simulink model "Model_2Systems_Manipulators"  (R2018b)
settings: Solver=ode23tb  StartTime=0.0  StopTime=10  RelTol=1e-3
values from neighbouring files (symbols this model uses):
  KL = [H_L1*TL(1:2,1:2) -H_L1 ; TL(3:4,1:2)+TL(3:4,3:4)*H_L1*TL(1:2,1:2) -TL(3:4,3:4)*H_L1]    [LaplaceScattering.m]    (also in SetScatteringGain.m)
  KR = [H_R1*TR(1:2,1:2) -H_R1 ; TR(3:4,1:2)+TR(3:4,3:4)*H_R1*TR(1:2,1:2) -TR(3:4,3:4)*H_R1]    [LaplaceScattering.m]    (also in SetScatteringGain.m)
  Kv = 0*eye(2)    [Parameters.m]
  p01 = zeros(SInfo1.n, 1)    [Parameters.m]
  p02 = zeros(SInfo2.n, 1)    [Parameters.m]
  q01 = [-pi;0.2;0.4]    [Parameters.m]
  q02 = [0.5; 1.5; pi/2+pi/4]    [Parameters.m]
  T12 = T    (= 0.1)    [Parameters.m]
  T21 = T*5    (= 0.5)    [Parameters.m]
  Vr0 = 0    [Parameters.m]
undefined symbols (not defined in the file or in its folder): Simulation
settings Model: Creator=oscar  LastModifiedBy=oscar
settings SolverCC: ZeroCrossAlgorithm=Adaptive
settings DataIOCC: OutputOption=SpecifiedOutputTimes  OutputTimes=t_out
settings SFSimCC: SimUseLocalCustomCode=off
settings RTWCC: RTWUseLocalCustomCode=off

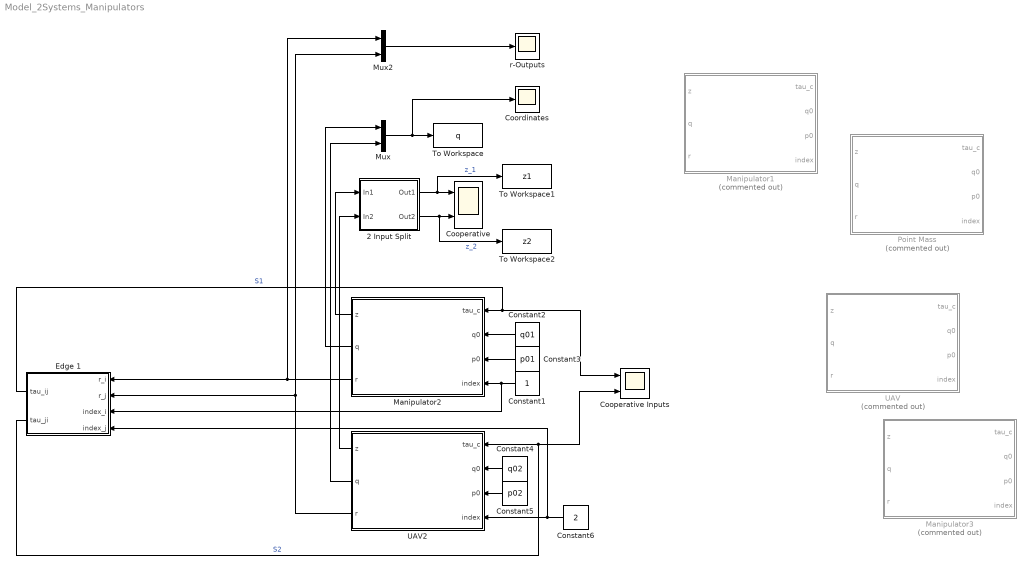
== system Model_2Systems_Manipulators ==
  2 Input Split : Subsystem
  Constant1 : Constant
  Constant2 : Constant  Value=q01
  Constant3 : Constant  Value=p01
  Constant4 : Constant  Value=q02
  Constant5 : Constant  Value=p02
  Constant6 : Constant  Value=2
  Cooperative : Scope  NumInputPorts=2
  Cooperative Inputs : Scope  NumInputPorts=2
  Coordinates : Scope
  Edge 1 : Subsystem
  Manipulator1 : Subsystem  Commented=on
  Manipulator2 : Subsystem
  Manipulator3 : Subsystem  Commented=on
  Mux : Mux  Inputs=2
  Mux2 : Mux  Inputs=2
  Point Mass : Subsystem  Commented=on
  To Workspace : ToWorkspace  VariableName=q  SaveFormat=Timeseries  SampleTime=-1
  To Workspace1 : ToWorkspace  VariableName=z1  SaveFormat=Timeseries  SampleTime=-1
  To Workspace2 : ToWorkspace  VariableName=z2  SaveFormat=Timeseries  SampleTime=-1
  UAV : Subsystem  Commented=on
  UAV2 : Subsystem
  r-Outputs : Scope
  wires:
  Mux/1 -> Coordinates/1, To Workspace/1
  Manipulator2/2(q) -> Mux/1
  UAV2/2(q) -> Mux/2
  Constant2/1 -> Manipulator2/2(q0)
  Constant3/1 -> Manipulator2/3(p0)
  Constant4/1 -> UAV2/2(q0)
  Constant5/1 -> UAV2/3(p0)
  Edge 1/1(tau_ij) -> Cooperative Inputs/1, Manipulator2/1(tau_c)  "S1"
  Edge 1/2(tau_ji) -> UAV2/1(tau_c), Cooperative Inputs/2  "S2"
  UAV2/3(r) -> Edge 1/2(r_j), Mux2/2
  Constant1/1 -> Manipulator2/4(index), Edge 1/3(index_i)
  Constant6/1 -> UAV2/4(index), Edge 1/4(index_j)
  Manipulator2/3(r) -> Edge 1/1(r_i), Mux2/1
  Mux2/1 -> r-Outputs/1
  Manipulator2/1(z) -> 2 Input Split/1(In1)
  UAV2/1(z) -> 2 Input Split/2(In2)
  2 Input Split/1(Out1) -> To Workspace1/1, Cooperative/1  "z_1"
  2 Input Split/2(Out2) -> To Workspace2/1, Cooperative/2  "z_2"

== system Model_2Systems_Manipulators/2 Input Split ==
  In1 : Inport
  In2 : Inport  Port=2
  Demux : Demux  Outputs=2
  Demux1 : Demux  Outputs=2
  Mux1 : Mux  Inputs=2
  Mux3 : Mux  Inputs=2
  Out1 : Outport
  Out2 : Outport  Port=2
  wires:
  Demux/1 -> Mux1/1
  Mux1/1 -> Out1/1
  In1/1 -> Demux/1
  Demux1/2 -> Mux3/2
  Mux3/1 -> Out2/1
  Demux1/1 -> Mux1/2
  Demux/2 -> Mux3/1
  In2/1 -> Demux1/1

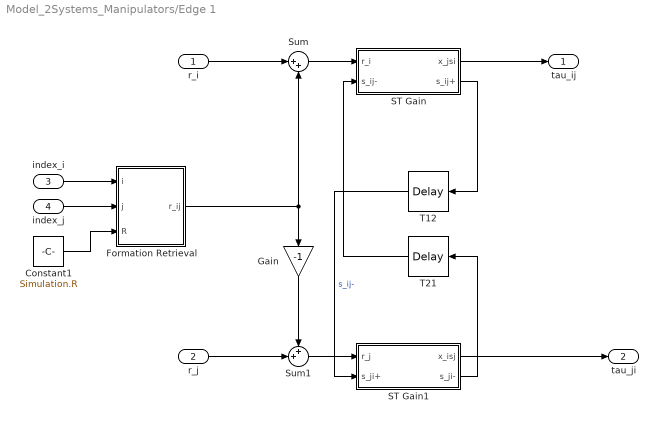
== system Model_2Systems_Manipulators/Edge 1 ==
  r_i : Inport
  r_j : Inport  Port=2
  index_i : Inport  Port=3
  index_j : Inport  Port=4
  Constant1 : Constant  Value=Simulation.R
  Formation Retrieval : MATLAB Function  TreatAsAtomicUnit=on
  Gain : Gain  Gain=-1
  ST Gain : Subsystem
  ST Gain1 : Subsystem
  Sum : Sum  Inputs=|++
  Sum1 : Sum  Inputs=++|
  T12 : TransportDelay  DelayTime=T12
  T21 : TransportDelay  DelayTime=T21
  tau_ij : Outport
  tau_ji : Outport  Port=2
  wires:
  r_i/1 -> Sum/1
  r_j/1 -> Sum1/2
  ST Gain/2(s_ij+) -> T12/1
  T21/1 -> ST Gain/2(s_ij-)
  T12/1 -> ST Gain1/2(s_ji+)  "s_ij-"
  ST Gain1/2(s_ji-) -> T21/1
  ST Gain/1(x_jsi) -> tau_ij/1
  ST Gain1/1(x_isj) -> tau_ji/1
  Sum/1 -> ST Gain/1(r_i)
  Sum1/1 -> ST Gain1/1(r_j)
  index_i/1 -> Formation Retrieval/1(i)
  index_j/1 -> Formation Retrieval/2(j)
  Formation Retrieval/1(r_ij) -> Gain/1, Sum/2
  Gain/1 -> Sum1/1
  Constant1/1 -> Formation Retrieval/3(R)

== system Model_2Systems_Manipulators/Manipulator1 ==
  tau_c : Inport
  q0 : Inport  Port=2
  p0 : Inport  Port=3
  index : Inport  Port=4
  Hamiltonian Plant : Subsystem
  Input Compensation : Scope  NumInputPorts=2
  Levenberg Compensation : MATLAB Function  Commented=on  TreatAsAtomicUnit=on
  Local Input : Scope
  MATLAB Function1 : MATLAB Function  TreatAsAtomicUnit=on
  Passivating Feedback : Scope
  Sum : Sum  Inputs=|++
  z : Outport
  q : Outport  Port=2
  r : Outport  Port=3
  wires:
  MATLAB Function1/1(tau) -> Hamiltonian Plant/3(tau_l), Local Input/1
  Hamiltonian Plant/4(p) -> MATLAB Function1/1(p)
  Hamiltonian Plant/3(q) -> q/1, MATLAB Function1/2(q)
  Hamiltonian Plant/5(z) -> z/1
  Hamiltonian Plant/2(r) -> r/1
  q0/1 -> Hamiltonian Plant/4(q0)
  p0/1 -> Hamiltonian Plant/5(p0)
  MATLAB Function1/2(tau_fb) -> Sum/2, Passivating Feedback/1
  index/1 -> Hamiltonian Plant/6(index), MATLAB Function1/3(index)
  Sum/1 -> Hamiltonian Plant/2(tau_c_hat), Input Compensation/2, Input Compensation/1  "tau_k"
  tau_c/1 -> Sum/1, Hamiltonian Plant/7(tau_c)  "tau_c_hat"

== system Model_2Systems_Manipulators/Manipulator2 ==
  tau_c : Inport
  q0 : Inport  Port=2
  p0 : Inport  Port=3
  index : Inport  Port=4
  Hamiltonian Plant : Subsystem
  Levenberg Compensation : MATLAB Function  Commented=on  TreatAsAtomicUnit=on
  Local Input : Scope
  MATLAB Function1 : MATLAB Function  TreatAsAtomicUnit=on
  Passivating Feedback : Scope
  Sum : Sum  Inputs=|++
  System Input : Scope
  z : Outport
  q : Outport  Port=2
  r : Outport  Port=3
  wires:
  MATLAB Function1/1(tau) -> Hamiltonian Plant/2(tau_l), Local Input/1
  Hamiltonian Plant/3(p) -> MATLAB Function1/1(p)
  Hamiltonian Plant/2(q) -> MATLAB Function1/2(q), q/1
  Hamiltonian Plant/4(z) -> z/1
  Hamiltonian Plant/1(r) -> r/1
  q0/1 -> Hamiltonian Plant/3(q0)
  p0/1 -> Hamiltonian Plant/4(p0)
  MATLAB Function1/2(tau_fb) -> Sum/2, Passivating Feedback/1
  index/1 -> Hamiltonian Plant/5(index), MATLAB Function1/3(index)
  Sum/1 -> Hamiltonian Plant/1(tau_c_hat), System Input/1  "tau_k"
  tau_c/1 -> Sum/1, Hamiltonian Plant/6(tau_c)  "tau_c_hat"

== system Model_2Systems_Manipulators/Manipulator3 ==
  note: z_dot Loop
  tau_c : Inport
  q0 : Inport  Port=2
  p0 : Inport  Port=3
  index : Inport  Port=4
  Gain : Gain  Gain=-Kv  Multiplication=Matrix(K*u)
  Hamiltonian Plant : Subsystem
  Input Compensation : Scope  NumInputPorts=2
  Levenberg Compensation : MATLAB Function  TreatAsAtomicUnit=on
  Local Input : Scope
  MATLAB Function1 : MATLAB Function  TreatAsAtomicUnit=on
  Passivating Feedback : Scope
  Sum : Sum  Inputs=|++
  z : Outport
  q : Outport  Port=2
  r : Outport  Port=3
  wires:
  MATLAB Function1/1(tau) -> Hamiltonian Plant/3(tau_l), Local Input/1
  Hamiltonian Plant/4(p) -> MATLAB Function1/1(p)
  Hamiltonian Plant/3(q) -> Levenberg Compensation/1(q), q/1, MATLAB Function1/2(q)
  Hamiltonian Plant/5(z) -> z/1
  Hamiltonian Plant/2(r) -> r/1
  q0/1 -> Hamiltonian Plant/4(q0)
  p0/1 -> Hamiltonian Plant/5(p0)
  MATLAB Function1/2(tau_fb) -> Sum/2, Passivating Feedback/1
  index/1 -> Levenberg Compensation/3(index), Hamiltonian Plant/6(index), MATLAB Function1/3(index)
  Hamiltonian Plant/1(z_dot) -> Gain/1
  Sum/1 -> Levenberg Compensation/2(tau_k), Input Compensation/1  "tau_k"
  tau_c/1 -> Sum/1, Hamiltonian Plant/7(tau_c)  "tau_c_hat"
  Levenberg Compensation/1(tau_c) -> Input Compensation/2, Hamiltonian Plant/2(tau_c_hat)  "tau_c_hat"

== system Model_2Systems_Manipulators/Point Mass ==
  tau_c : Inport
  q0 : Inport  Port=2
  p0 : Inport  Port=3
  index : Inport  Port=4
  Hamiltonian Plant : Subsystem
  MATLAB Function1 : MATLAB Function  TreatAsAtomicUnit=on
  Scope : Scope
  Sum : Sum  Inputs=|++
  z : Outport
  q : Outport  Port=2
  r : Outport  Port=3
  wires:
  MATLAB Function1/1(tau) -> Hamiltonian Plant/2(tau_l)
  tau_c/1 -> Sum/1
  Hamiltonian Plant/3(p) -> MATLAB Function1/1(p)
  Hamiltonian Plant/2(q) -> MATLAB Function1/2(q), q/1
  Hamiltonian Plant/4(z) -> z/1
  Hamiltonian Plant/1(r) -> r/1
  q0/1 -> Hamiltonian Plant/3(q0)
  p0/1 -> Hamiltonian Plant/4(p0)
  MATLAB Function1/2(tau_fb) -> Scope/1, Sum/2
  Sum/1 -> Hamiltonian Plant/1(tau_c)
  index/1 -> Hamiltonian Plant/5(index), MATLAB Function1/3(index)

== system Model_2Systems_Manipulators/UAV ==
  tau_c : Inport
  q0 : Inport  Port=2
  p0 : Inport  Port=3
  index : Inport  Port=4
  Gain : Gain  Gain=Kv  Multiplication=Matrix(K*u)
  Hamiltonian Plant : Subsystem
  MATLAB Function1 : MATLAB Function  TreatAsAtomicUnit=on
  Scope : Scope
  Scope1 : Scope
  Sum : Sum  Inputs=|++
  Sum1 : Sum  Inputs=-+|
  z : Outport
  q : Outport  Port=2
  r : Outport  Port=3
  wires:
  MATLAB Function1/1(tau) -> Scope1/1, Hamiltonian Plant/2(tau_l)
  tau_c/1 -> Sum/1
  Hamiltonian Plant/3(p) -> MATLAB Function1/1(p)
  Hamiltonian Plant/2(q) -> MATLAB Function1/2(q), q/1
  Hamiltonian Plant/4(z) -> z/1
  Hamiltonian Plant/1(r) -> r/1
  q0/1 -> Hamiltonian Plant/3(q0)
  p0/1 -> Hamiltonian Plant/4(p0)
  MATLAB Function1/2(tau_fb) -> Scope/1, Sum/2
  Sum/1 -> Sum1/2
  index/1 -> Hamiltonian Plant/5(index), MATLAB Function1/3(index)
  Hamiltonian Plant/5(y) -> Gain/1
  Sum1/1 -> Hamiltonian Plant/1(tau_c)
  Gain/1 -> Sum1/1

== system Model_2Systems_Manipulators/UAV2 ==
  tau_c : Inport
  q0 : Inport  Port=2
  p0 : Inport  Port=3
  index : Inport  Port=4
  Hamiltonian Plant : Subsystem
  Levenberg Compensation : MATLAB Function  Commented=on  TreatAsAtomicUnit=on
  Local Input : Scope
  MATLAB Function : MATLAB Function  TreatAsAtomicUnit=on
  MATLAB Function1 : MATLAB Function  Commented=on  TreatAsAtomicUnit=on
  Passivating Feedback : Scope
  Sum : Sum  Inputs=|++
  System Input : Scope
  z : Outport
  q : Outport  Port=2
  r : Outport  Port=3
  wires:
  ? -> Hamiltonian Plant/2(tau_l), Local Input/1
  Hamiltonian Plant/3(p) -> ?
  Hamiltonian Plant/2(q) -> q/1
  Hamiltonian Plant/4(z) -> z/1
  Hamiltonian Plant/1(r) -> r/1
  q0/1 -> Hamiltonian Plant/3(q0)
  p0/1 -> Hamiltonian Plant/4(p0)
  ? -> Sum/2, Passivating Feedback/1
  index/1 -> Hamiltonian Plant/5(index)
  Sum/1 -> Hamiltonian Plant/1(tau_c_hat), System Input/1  "tau_c_hat"
  tau_c/1 -> Sum/1, Hamiltonian Plant/6(tau_c)

== system Model_2Systems_Manipulators/Edge 1/ST Gain ==
  r_i : Inport
  s_ij- : Inport  Port=2
  Demux : Demux  Outputs=2
  Gain : Gain  Gain=KL  Multiplication=Matrix(K*u)
  Mux : Mux  Inputs=2
  x_jsi : Outport
  s_ij+ : Outport  Port=2
  wires:
  s_ij-/1 -> Mux/1
  r_i/1 -> Mux/2
  Mux/1 -> Gain/1
  Gain/1 -> Demux/1
  Demux/1 -> x_jsi/1
  Demux/2 -> s_ij+/1

== system Model_2Systems_Manipulators/Edge 1/ST Gain1 ==
  r_j : Inport
  s_ji+ : Inport  Port=2
  Demux : Demux  Outputs=2
  Gain : Gain  Gain=KR  Multiplication=Matrix(K*u)
  Mux : Mux  Inputs=2
  x_isj : Outport
  s_ji- : Outport  Port=2
  wires:
  s_ji+/1 -> Mux/1
  r_j/1 -> Mux/2
  Mux/1 -> Gain/1
  Gain/1 -> Demux/1
  Demux/1 -> x_isj/1
  Demux/2 -> s_ji-/1

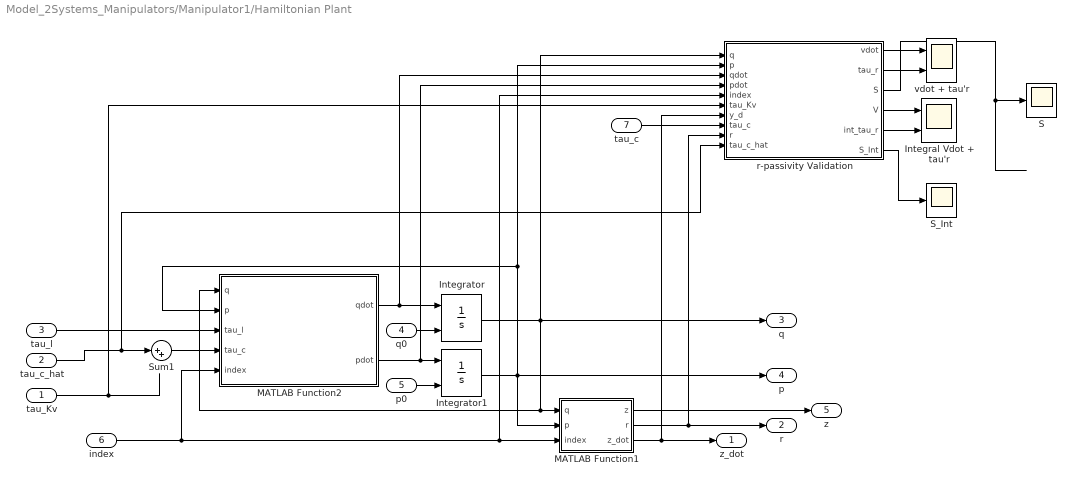
== system Model_2Systems_Manipulators/Manipulator1/Hamiltonian Plant ==
  tau_Kv : Inport
  tau_c_hat : Inport  Port=2
  tau_l : Inport  Port=3
  q0 : Inport  Port=4
  p0 : Inport  Port=5
  index : Inport  Port=6
  tau_c : Inport  Port=7
  Integral Vdot + tau'r : Scope  NumInputPorts=2
  Integrator : Integrator  InitialConditionSource=external  InitialCondition=q01
  Integrator1 : Integrator  InitialConditionSource=external  InitialCondition=p02
  MATLAB Function1 : MATLAB Function  TreatAsAtomicUnit=on
  MATLAB Function2 : MATLAB Function  TreatAsAtomicUnit=on
  S : Scope
  S_Int : Scope
  Sum1 : Sum  Inputs=|++
  r-passivity Validation : Subsystem
  vdot + tau'r : Scope  NumInputPorts=2
  z_dot : Outport
  r : Outport  Port=2
  q : Outport  Port=3
  p : Outport  Port=4
  z : Outport  Port=5
  wires:
  tau_l/1 -> MATLAB Function2/3(tau_l)
  MATLAB Function2/2(pdot) -> r-passivity Validation/4(pdot), Integrator1/1
  Integrator1/1 -> r-passivity Validation/2(p), MATLAB Function2/2(p), p/1, MATLAB Function1/2(p)
  Integrator/1 -> r-passivity Validation/1(q), q/1, MATLAB Function2/1(q), MATLAB Function1/1(q)
  MATLAB Function2/1(qdot) -> r-passivity Validation/3(qdot), Integrator/1
  p0/1 -> Integrator1/2
  tau_c_hat/1 -> r-passivity Validation/10(tau_c_hat), Sum1/1
  q0/1 -> Integrator/2
  MATLAB Function1/1(z) -> z/1
  MATLAB Function1/2(r) -> r-passivity Validation/9(r), r/1
  index/1 -> r-passivity Validation/5(index), MATLAB Function1/3(index), MATLAB Function2/5(index)
  MATLAB Function1/3(z_dot) -> r-passivity Validation/7(y_d), z_dot/1
  r-passivity Validation/1(vdot) -> vdot + tau'r/1
  r-passivity Validation/2(tau_r) -> vdot + tau'r/2
  r-passivity Validation/5(int_tau_r) -> Integral Vdot + tau'r/2
  r-passivity Validation/4(V) -> Integral Vdot + tau'r/1
  r-passivity Validation/3(S) -> S/1
  tau_c/1 -> r-passivity Validation/8(tau_c)
  tau_Kv/1 -> r-passivity Validation/6(tau_Kv)
  Sum1/1 -> MATLAB Function2/4(tau_c)
  r-passivity Validation/6(S_Int) -> S_Int/1

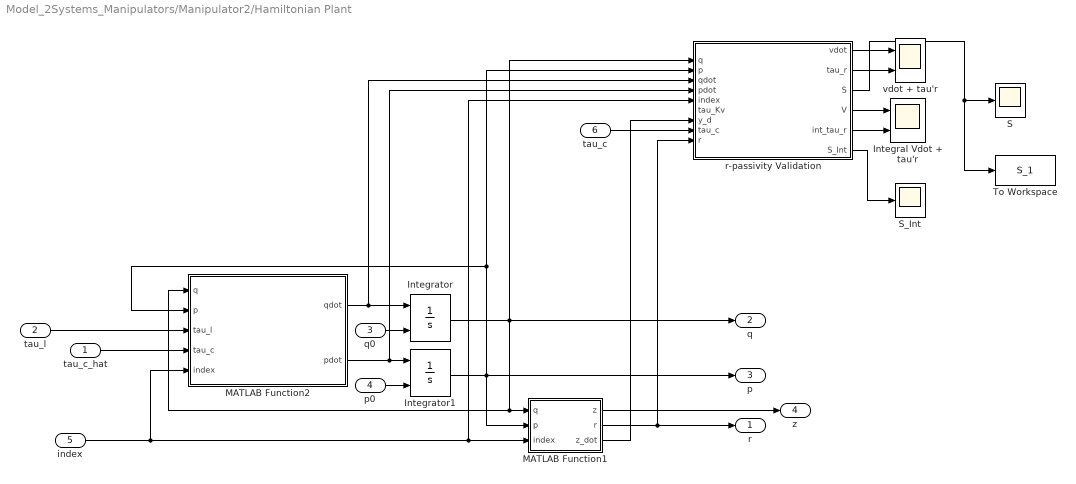
== system Model_2Systems_Manipulators/Manipulator2/Hamiltonian Plant ==
  tau_c_hat : Inport
  tau_l : Inport  Port=2
  q0 : Inport  Port=3
  p0 : Inport  Port=4
  index : Inport  Port=5
  tau_c : Inport  Port=6
  Integral Vdot + tau'r : Scope  NumInputPorts=2
  Integrator : Integrator  InitialConditionSource=external  InitialCondition=q01
  Integrator1 : Integrator  InitialConditionSource=external  InitialCondition=p02
  MATLAB Function1 : MATLAB Function  TreatAsAtomicUnit=on
  MATLAB Function2 : MATLAB Function  TreatAsAtomicUnit=on
  S : Scope
  S_Int : Scope
  To Workspace : ToWorkspace  VariableName=S_1  SaveFormat=Timeseries  SampleTime=-1
  r-passivity Validation : Subsystem
  vdot + tau'r : Scope  NumInputPorts=2
  r : Outport
  q : Outport  Port=2
  p : Outport  Port=3
  z : Outport  Port=4
  wires:
  tau_l/1 -> MATLAB Function2/3(tau_l)
  MATLAB Function2/2(pdot) -> r-passivity Validation/4(pdot), Integrator1/1
  Integrator1/1 -> r-passivity Validation/2(p), MATLAB Function2/2(p), p/1, MATLAB Function1/2(p)
  Integrator/1 -> r-passivity Validation/1(q), q/1, MATLAB Function2/1(q), MATLAB Function1/1(q)
  MATLAB Function2/1(qdot) -> r-passivity Validation/3(qdot), Integrator/1
  p0/1 -> Integrator1/2
  q0/1 -> Integrator/2
  MATLAB Function1/1(z) -> z/1
  MATLAB Function1/2(r) -> r-passivity Validation/9(r), r/1
  index/1 -> r-passivity Validation/5(index), MATLAB Function1/3(index), MATLAB Function2/5(index)
  MATLAB Function1/3(z_dot) -> r-passivity Validation/7(y_d)
  r-passivity Validation/1(vdot) -> vdot + tau'r/1
  r-passivity Validation/2(tau_r) -> vdot + tau'r/2
  r-passivity Validation/5(int_tau_r) -> Integral Vdot + tau'r/2
  r-passivity Validation/4(V) -> Integral Vdot + tau'r/1
  r-passivity Validation/3(S) -> To Workspace/1, S/1
  tau_c/1 -> r-passivity Validation/8(tau_c)
  tau_c_hat/1 -> MATLAB Function2/4(tau_c)
  r-passivity Validation/6(S_Int) -> S_Int/1

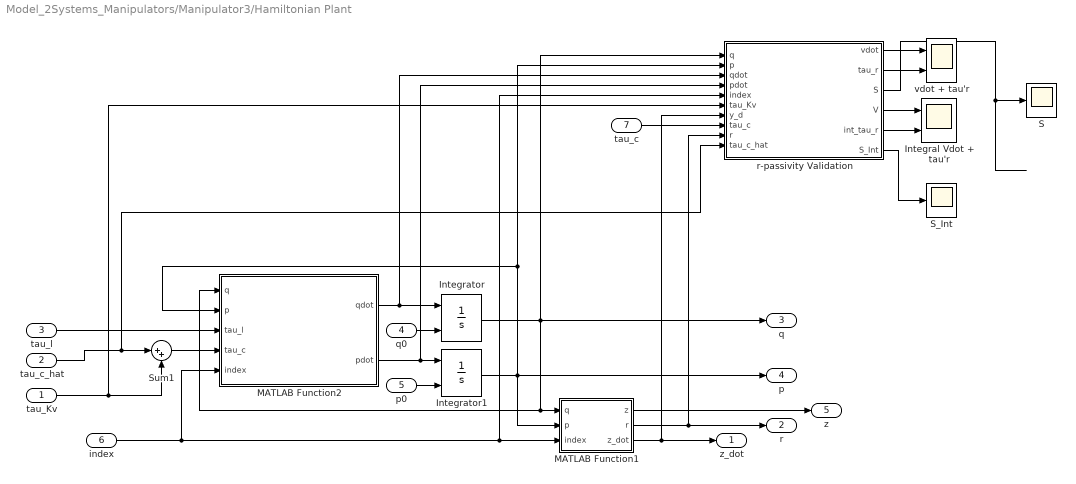
== system Model_2Systems_Manipulators/Manipulator3/Hamiltonian Plant ==
  tau_Kv : Inport
  tau_c_hat : Inport  Port=2
  tau_l : Inport  Port=3
  q0 : Inport  Port=4
  p0 : Inport  Port=5
  index : Inport  Port=6
  tau_c : Inport  Port=7
  Integral Vdot + tau'r : Scope  NumInputPorts=2
  Integrator : Integrator  InitialConditionSource=external  InitialCondition=q01
  Integrator1 : Integrator  InitialConditionSource=external  InitialCondition=p02
  MATLAB Function1 : MATLAB Function  TreatAsAtomicUnit=on
  MATLAB Function2 : MATLAB Function  TreatAsAtomicUnit=on
  S : Scope
  S_Int : Scope
  Sum1 : Sum  Inputs=|++
  r-passivity Validation : Subsystem
  vdot + tau'r : Scope  NumInputPorts=2
  z_dot : Outport
  r : Outport  Port=2
  q : Outport  Port=3
  p : Outport  Port=4
  z : Outport  Port=5
  wires:
  tau_l/1 -> MATLAB Function2/3(tau_l)
  MATLAB Function2/2(pdot) -> r-passivity Validation/4(pdot), Integrator1/1
  Integrator1/1 -> r-passivity Validation/2(p), MATLAB Function2/2(p), p/1, MATLAB Function1/2(p)
  Integrator/1 -> r-passivity Validation/1(q), q/1, MATLAB Function2/1(q), MATLAB Function1/1(q)
  MATLAB Function2/1(qdot) -> r-passivity Validation/3(qdot), Integrator/1
  p0/1 -> Integrator1/2
  tau_c_hat/1 -> r-passivity Validation/10(tau_c_hat), Sum1/1
  q0/1 -> Integrator/2
  MATLAB Function1/1(z) -> z/1
  MATLAB Function1/2(r) -> r-passivity Validation/9(r), r/1
  index/1 -> r-passivity Validation/5(index), MATLAB Function1/3(index), MATLAB Function2/5(index)
  MATLAB Function1/3(z_dot) -> r-passivity Validation/7(y_d), z_dot/1
  r-passivity Validation/1(vdot) -> vdot + tau'r/1
  r-passivity Validation/2(tau_r) -> vdot + tau'r/2
  r-passivity Validation/5(int_tau_r) -> Integral Vdot + tau'r/2
  r-passivity Validation/4(V) -> Integral Vdot + tau'r/1
  r-passivity Validation/3(S) -> S/1
  tau_c/1 -> r-passivity Validation/8(tau_c)
  tau_Kv/1 -> Sum1/2, r-passivity Validation/6(tau_Kv)
  Sum1/1 -> MATLAB Function2/4(tau_c)
  r-passivity Validation/6(S_Int) -> S_Int/1

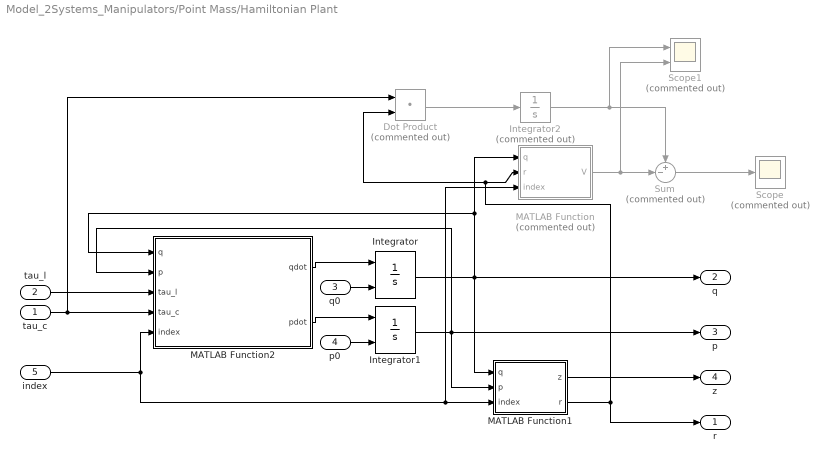
== system Model_2Systems_Manipulators/Point Mass/Hamiltonian Plant ==
  tau_c : Inport
  tau_l : Inport  Port=2
  q0 : Inport  Port=3
  p0 : Inport  Port=4
  index : Inport  Port=5
  Dot Product : DotProduct  Commented=on  InputSameDT=on  OutDataTypeStr=Inherit: Inherit via internal rule
  Integrator : Integrator  InitialConditionSource=external  InitialCondition=q01
  Integrator1 : Integrator  InitialConditionSource=external  InitialCondition=p02
  Integrator2 : Integrator  Commented=on
  MATLAB Function : MATLAB Function  Commented=on  TreatAsAtomicUnit=on
  MATLAB Function1 : MATLAB Function  TreatAsAtomicUnit=on
  MATLAB Function2 : MATLAB Function  TreatAsAtomicUnit=on
  Scope : Scope  Commented=on
  Scope1 : Scope  Commented=on  NumInputPorts=2
  Sum : Sum  Commented=on  Inputs=+-|
  r : Outport
  q : Outport  Port=2
  p : Outport  Port=3
  z : Outport  Port=4
  wires:
  tau_l/1 -> MATLAB Function2/3(tau_l)
  MATLAB Function2/2(pdot) -> Integrator1/1
  Integrator1/1 -> MATLAB Function1/2(p), MATLAB Function2/2(p), p/1
  Integrator/1 -> MATLAB Function1/1(q), MATLAB Function/1(q), MATLAB Function2/1(q), q/1
  MATLAB Function2/1(qdot) -> Integrator/1
  p0/1 -> Integrator1/2
  tau_c/1 -> MATLAB Function2/4(tau_c), Dot Product/1
  q0/1 -> Integrator/2
  MATLAB Function/1(V) -> Scope1/2, Sum/2
  Dot Product/1 -> Integrator2/1
  Sum/1 -> Scope/1
  Integrator2/1 -> Scope1/1, Sum/1
  MATLAB Function1/1(z) -> z/1
  MATLAB Function1/2(r) -> MATLAB Function/2(r), Dot Product/2, r/1
  index/1 -> MATLAB Function/3(index), MATLAB Function1/3(index), MATLAB Function2/5(index)

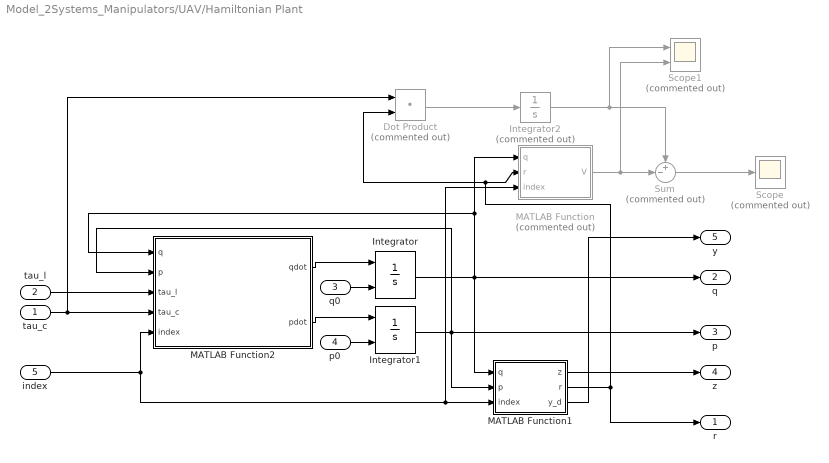
== system Model_2Systems_Manipulators/UAV/Hamiltonian Plant ==
  tau_c : Inport
  tau_l : Inport  Port=2
  q0 : Inport  Port=3
  p0 : Inport  Port=4
  index : Inport  Port=5
  Dot Product : DotProduct  Commented=on  InputSameDT=on  OutDataTypeStr=Inherit: Inherit via internal rule
  Integrator : Integrator  InitialConditionSource=external  InitialCondition=q01
  Integrator1 : Integrator  InitialConditionSource=external  InitialCondition=p02
  Integrator2 : Integrator  Commented=on
  MATLAB Function : MATLAB Function  Commented=on  TreatAsAtomicUnit=on
  MATLAB Function1 : MATLAB Function  TreatAsAtomicUnit=on
  MATLAB Function2 : MATLAB Function  TreatAsAtomicUnit=on
  Scope : Scope  Commented=on
  Scope1 : Scope  Commented=on  NumInputPorts=2
  Sum : Sum  Commented=on  Inputs=+-|
  r : Outport
  q : Outport  Port=2
  p : Outport  Port=3
  z : Outport  Port=4
  y : Outport  Port=5
  wires:
  tau_l/1 -> MATLAB Function2/3(tau_l)
  MATLAB Function2/2(pdot) -> Integrator1/1
  Integrator1/1 -> MATLAB Function1/2(p), MATLAB Function2/2(p), p/1
  Integrator/1 -> MATLAB Function1/1(q), MATLAB Function/1(q), MATLAB Function2/1(q), q/1
  MATLAB Function2/1(qdot) -> Integrator/1
  p0/1 -> Integrator1/2
  tau_c/1 -> MATLAB Function2/4(tau_c), Dot Product/1
  q0/1 -> Integrator/2
  MATLAB Function/1(V) -> Scope1/2, Sum/2
  Dot Product/1 -> Integrator2/1
  Sum/1 -> Scope/1
  Integrator2/1 -> Scope1/1, Sum/1
  MATLAB Function1/1(z) -> z/1
  MATLAB Function1/2(r) -> r/1, MATLAB Function/2(r), Dot Product/2
  index/1 -> MATLAB Function/3(index), MATLAB Function1/3(index), MATLAB Function2/5(index)
  MATLAB Function1/3(y_d) -> y/1

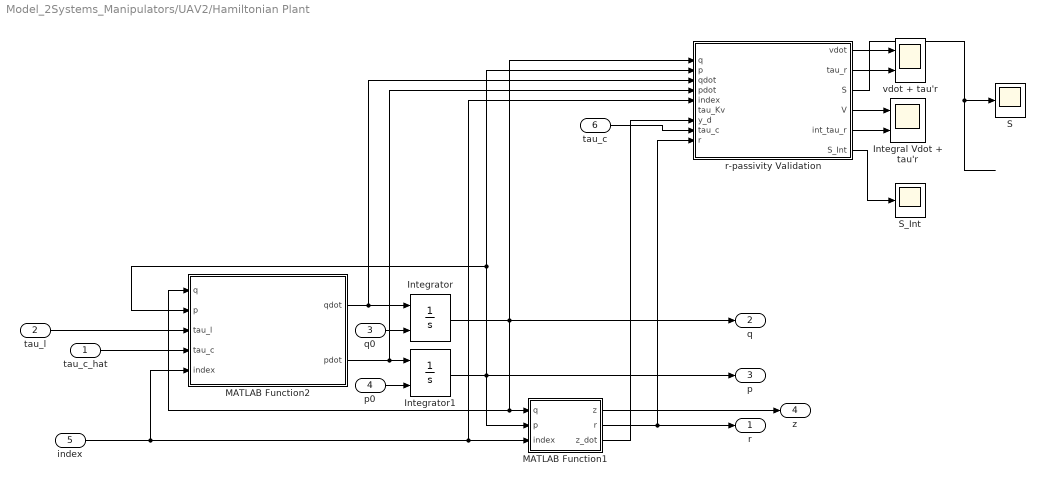
== system Model_2Systems_Manipulators/UAV2/Hamiltonian Plant ==
  tau_c_hat : Inport
  tau_l : Inport  Port=2
  q0 : Inport  Port=3
  p0 : Inport  Port=4
  index : Inport  Port=5
  tau_c : Inport  Port=6
  Integral Vdot + tau'r : Scope  NumInputPorts=2
  Integrator : Integrator  InitialConditionSource=external  InitialCondition=q01
  Integrator1 : Integrator  InitialConditionSource=external  InitialCondition=p02
  MATLAB Function1 : MATLAB Function  TreatAsAtomicUnit=on
  MATLAB Function2 : MATLAB Function  TreatAsAtomicUnit=on
  S : Scope
  S_Int : Scope
  r-passivity Validation : Subsystem
  vdot + tau'r : Scope  NumInputPorts=2
  r : Outport
  q : Outport  Port=2
  p : Outport  Port=3
  z : Outport  Port=4
  wires:
  tau_l/1 -> MATLAB Function2/3(tau_l)
  MATLAB Function2/2(pdot) -> r-passivity Validation/4(pdot), Integrator1/1
  Integrator1/1 -> r-passivity Validation/2(p), MATLAB Function2/2(p), p/1, MATLAB Function1/2(p)
  Integrator/1 -> r-passivity Validation/1(q), q/1, MATLAB Function2/1(q), MATLAB Function1/1(q)
  MATLAB Function2/1(qdot) -> r-passivity Validation/3(qdot), Integrator/1
  p0/1 -> Integrator1/2
  q0/1 -> Integrator/2
  MATLAB Function1/1(z) -> z/1
  MATLAB Function1/2(r) -> r-passivity Validation/9(r), r/1
  index/1 -> r-passivity Validation/5(index), MATLAB Function1/3(index), MATLAB Function2/5(index)
  MATLAB Function1/3(z_dot) -> r-passivity Validation/7(y_d)
  r-passivity Validation/1(vdot) -> vdot + tau'r/1
  r-passivity Validation/2(tau_r) -> vdot + tau'r/2
  r-passivity Validation/5(int_tau_r) -> Integral Vdot + tau'r/2
  r-passivity Validation/4(V) -> Integral Vdot + tau'r/1
  r-passivity Validation/3(S) -> S/1
  tau_c/1 -> r-passivity Validation/8(tau_c)
  tau_c_hat/1 -> MATLAB Function2/4(tau_c)
  r-passivity Validation/6(S_Int) -> S_Int/1

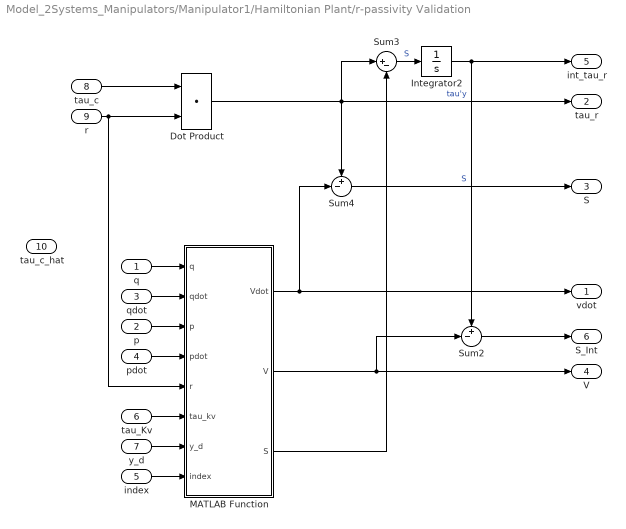
== system Model_2Systems_Manipulators/Manipulator1/Hamiltonian Plant/r-passivity Validation ==
  q : Inport
  p : Inport  Port=2
  qdot : Inport  Port=3
  pdot : Inport  Port=4
  index : Inport  Port=5
  tau_Kv : Inport  Port=6
  y_d : Inport  Port=7
  tau_c : Inport  Port=8
  r : Inport  Port=9
  tau_c_hat : Inport  Port=10
  Dot Product : DotProduct  InputSameDT=on  OutDataTypeStr=Inherit: Inherit via internal rule
  Integrator2 : Integrator
  MATLAB Function : MATLAB Function  TreatAsAtomicUnit=on
  Sum2 : Sum  Inputs=+-|
  Sum3 : Sum  Inputs=|+-
  Sum4 : Sum  Inputs=+-|
  vdot : Outport
  tau_r : Outport  Port=2
  S : Outport  Port=3
  V : Outport  Port=4
  int_tau_r : Outport  Port=5
  S_Int : Outport  Port=6
  wires:
  Sum4/1 -> S/1  "S"
  pdot/1 -> MATLAB Function/4(pdot)
  p/1 -> MATLAB Function/3(p)
  qdot/1 -> MATLAB Function/2(qdot)
  index/1 -> MATLAB Function/8(index)
  q/1 -> MATLAB Function/1(q)
  tau_Kv/1 -> MATLAB Function/6(tau_kv)
  y_d/1 -> MATLAB Function/7(y_d)
  tau_c/1 -> Dot Product/1
  r/1 -> Dot Product/2, MATLAB Function/5(r)
  Dot Product/1 -> Sum3/1, tau_r/1, Sum4/1  "tau'y"
  MATLAB Function/1(Vdot) -> Sum4/2, vdot/1
  MATLAB Function/2(V) -> Sum2/2, V/1
  Integrator2/1 -> int_tau_r/1, Sum2/1
  Sum2/1 -> S_Int/1
  MATLAB Function/3(S) -> Sum3/2
  Sum3/1 -> Integrator2/1  "S"

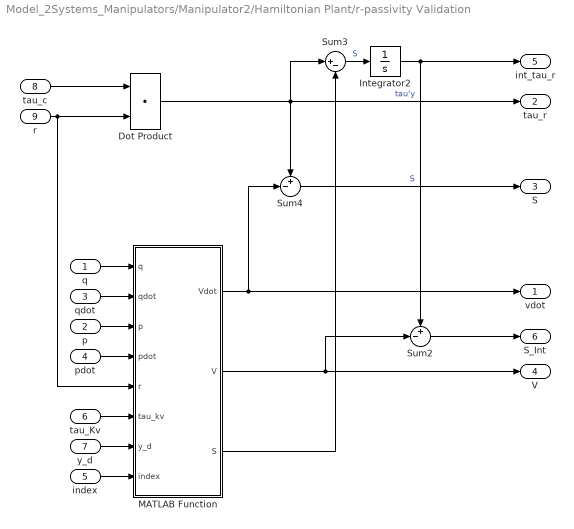
== system Model_2Systems_Manipulators/Manipulator2/Hamiltonian Plant/r-passivity Validation ==
  q : Inport
  p : Inport  Port=2
  qdot : Inport  Port=3
  pdot : Inport  Port=4
  index : Inport  Port=5
  tau_Kv : Inport  Port=6
  y_d : Inport  Port=7
  tau_c : Inport  Port=8
  r : Inport  Port=9
  Dot Product : DotProduct  InputSameDT=on  OutDataTypeStr=Inherit: Inherit via internal rule
  Integrator2 : Integrator
  MATLAB Function : MATLAB Function  TreatAsAtomicUnit=on
  Sum2 : Sum  Inputs=+-|
  Sum3 : Sum  Inputs=|+-
  Sum4 : Sum  Inputs=+-|
  vdot : Outport
  tau_r : Outport  Port=2
  S : Outport  Port=3
  V : Outport  Port=4
  int_tau_r : Outport  Port=5
  S_Int : Outport  Port=6
  wires:
  Sum4/1 -> S/1  "S"
  pdot/1 -> MATLAB Function/4(pdot)
  p/1 -> MATLAB Function/3(p)
  qdot/1 -> MATLAB Function/2(qdot)
  index/1 -> MATLAB Function/8(index)
  q/1 -> MATLAB Function/1(q)
  tau_Kv/1 -> MATLAB Function/6(tau_kv)
  y_d/1 -> MATLAB Function/7(y_d)
  tau_c/1 -> Dot Product/1
  r/1 -> Dot Product/2, MATLAB Function/5(r)
  Dot Product/1 -> Sum3/1, tau_r/1, Sum4/1  "tau'y"
  MATLAB Function/1(Vdot) -> Sum4/2, vdot/1
  MATLAB Function/2(V) -> Sum2/2, V/1
  Integrator2/1 -> int_tau_r/1, Sum2/1
  Sum2/1 -> S_Int/1
  MATLAB Function/3(S) -> Sum3/2
  Sum3/1 -> Integrator2/1  "S"

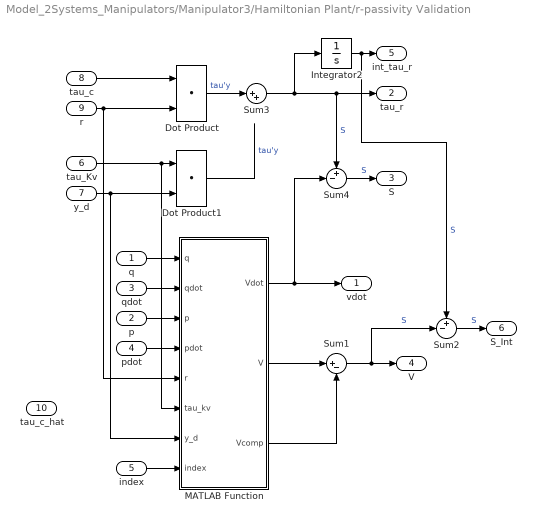
== system Model_2Systems_Manipulators/Manipulator3/Hamiltonian Plant/r-passivity Validation ==
  q : Inport
  p : Inport  Port=2
  qdot : Inport  Port=3
  pdot : Inport  Port=4
  index : Inport  Port=5
  tau_Kv : Inport  Port=6
  y_d : Inport  Port=7
  tau_c : Inport  Port=8
  r : Inport  Port=9
  tau_c_hat : Inport  Port=10
  Dot Product : DotProduct  InputSameDT=on  OutDataTypeStr=Inherit: Inherit via internal rule
  Dot Product1 : DotProduct  InputSameDT=on  OutDataTypeStr=Inherit: Inherit via internal rule
  Integrator2 : Integrator
  MATLAB Function : MATLAB Function  TreatAsAtomicUnit=on
  Sum1 : Sum  Inputs=|+-
  Sum2 : Sum  Inputs=+-|
  Sum3 : Sum  Inputs=|++
  Sum4 : Sum  Inputs=+-|
  vdot : Outport
  tau_r : Outport  Port=2
  S : Outport  Port=3
  V : Outport  Port=4
  int_tau_r : Outport  Port=5
  S_Int : Outport  Port=6
  wires:
  Sum4/1 -> S/1  "S"
  pdot/1 -> MATLAB Function/4(pdot)
  p/1 -> MATLAB Function/3(p)
  qdot/1 -> MATLAB Function/2(qdot)
  MATLAB Function/2(V) -> Sum1/1
  index/1 -> MATLAB Function/8(index)
  q/1 -> MATLAB Function/1(q)
  tau_Kv/1 -> MATLAB Function/6(tau_kv), Dot Product1/1
  y_d/1 -> Dot Product1/2, MATLAB Function/7(y_d)
  tau_c/1 -> Dot Product/1
  r/1 -> Dot Product/2, MATLAB Function/5(r)
  Dot Product/1 -> Sum3/1  "tau'y"
  Sum3/1 -> Integrator2/1, tau_r/1, Sum4/1  "S"
  Dot Product1/1 -> ?  "tau'y"
  MATLAB Function/1(Vdot) -> Sum4/2, vdot/1
  Sum1/1 -> Sum2/2, V/1  "S"
  MATLAB Function/3(Vcomp) -> Sum1/2
  Integrator2/1 -> Sum2/1, int_tau_r/1  "S"
  Sum2/1 -> S_Int/1  "S"

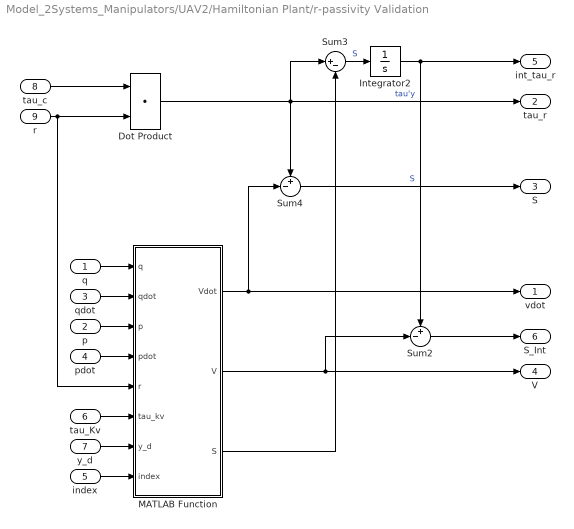
== system Model_2Systems_Manipulators/UAV2/Hamiltonian Plant/r-passivity Validation ==
  q : Inport
  p : Inport  Port=2
  qdot : Inport  Port=3
  pdot : Inport  Port=4
  index : Inport  Port=5
  tau_Kv : Inport  Port=6
  y_d : Inport  Port=7
  tau_c : Inport  Port=8
  r : Inport  Port=9
  Dot Product : DotProduct  InputSameDT=on  OutDataTypeStr=Inherit: Inherit via internal rule
  Integrator2 : Integrator
  MATLAB Function : MATLAB Function  TreatAsAtomicUnit=on
  Sum2 : Sum  Inputs=+-|
  Sum3 : Sum  Inputs=|+-
  Sum4 : Sum  Inputs=+-|
  vdot : Outport
  tau_r : Outport  Port=2
  S : Outport  Port=3
  V : Outport  Port=4
  int_tau_r : Outport  Port=5
  S_Int : Outport  Port=6
  wires:
  Sum4/1 -> S/1  "S"
  pdot/1 -> MATLAB Function/4(pdot)
  p/1 -> MATLAB Function/3(p)
  qdot/1 -> MATLAB Function/2(qdot)
  index/1 -> MATLAB Function/8(index)
  q/1 -> MATLAB Function/1(q)
  tau_Kv/1 -> MATLAB Function/6(tau_kv)
  y_d/1 -> MATLAB Function/7(y_d)
  tau_c/1 -> Dot Product/1
  r/1 -> Dot Product/2, MATLAB Function/5(r)
  Dot Product/1 -> Sum3/1, tau_r/1, Sum4/1  "tau'y"
  MATLAB Function/1(Vdot) -> Sum4/2, vdot/1
  MATLAB Function/2(V) -> Sum2/2, V/1
  Integrator2/1 -> int_tau_r/1, Sum2/1
  Sum2/1 -> S_Int/1
  MATLAB Function/3(S) -> Sum3/2
  Sum3/1 -> Integrator2/1  "S"

== matlab function Model_2Systems_Manipulators/Point Mass/Hamiltonian Plant/MATLAB Function ==
  data: q input; r input; index input; V output; Vr0 parameter
function V = fcn(q, r, index, Vr0)

%     coder.extrinsic('R_Validation');
%     V = 0;
%     [V] = R_Validation(q, r, index);
%     V = V - Vr0;
V = 0;
end

== matlab function Model_2Systems_Manipulators/Point Mass/Hamiltonian Plant/MATLAB Function1 ==
  data: q input; z output; p input; r output; index input
function [z, r] = toz(q, p, index)

    coder.extrinsic('Pointmass2D_z');
    z = zeros(2, 1);
    r = zeros(2, 1);    
    [z, r] = Pointmass2D_z(q, p, index);

== matlab function Model_2Systems_Manipulators/Manipulator2/Hamiltonian Plant/MATLAB Function1 ==
  data: q input; z output; p input; r output; index input; z_dot output
function [z, r, z_dot] = toz(q, p, index)

    coder.extrinsic('Manipulator_z');
    z = zeros(2, 1);
    r = zeros(2, 1);
    z_dot = zeros(2, 1);
    [z, r, z_dot] = Manipulator_z(q, p, index);

== matlab function Model_2Systems_Manipulators/Manipulator2/Hamiltonian Plant/MATLAB Function2 ==
  data: q input; qdot output; p input; tau_l input; pdot output; tau_c input; index input
function [qdot, pdot] = fcn(q, p, tau_l, tau_c, index)

    coder.extrinsic('Manipulator_Dynamics');
    qdot = zeros(3, 1);
    pdot = zeros(3, 1);
    [qdot, pdot] = Manipulator_Dynamics(q, p, tau_l, tau_c, index);

== matlab function Model_2Systems_Manipulators/Point Mass/Hamiltonian Plant/MATLAB Function2 ==
  data: q input; qdot output; p input; tau_l input; pdot output; tau_c input; index input
function [qdot, pdot] = fcn(q, p, tau_l, tau_c, index)

    coder.extrinsic('Pointmass2D_Dynamics');
    qdot = zeros(2, 1);
    pdot = zeros(2, 1);
    [qdot, pdot] = Pointmass2D_Dynamics(q, p, tau_l, tau_c, index);

== matlab function Model_2Systems_Manipulators/Point Mass/MATLAB Function1 ==
  data: p input; q input; tau output; tau_fb output; index input
function [tau, tau_fb] = LocalControl(p, q, index)
    

coder.extrinsic('Pointmass2D_Control');
tau = zeros(2, 1);
tau_fb = zeros(2, 1);
[tau, tau_fb] = Pointmass2D_Control(q, p, index);

== matlab function Model_2Systems_Manipulators/Manipulator1/Hamiltonian Plant/MATLAB Function1 ==
  data: q input; z output; p input; r output; index input; z_dot output
function [z, r, z_dot] = toz(q, p, index)

    coder.extrinsic('Manipulator_z');
    z = zeros(2, 1);
    r = zeros(2, 1);
    z_dot = zeros(2, 1);
    [z, r, z_dot] = Manipulator_z(q, p, index);

== matlab function Model_2Systems_Manipulators/Manipulator1/Hamiltonian Plant/MATLAB Function2 ==
  data: q input; qdot output; p input; tau_l input; pdot output; tau_c input; index input
function [qdot, pdot] = fcn(q, p, tau_l, tau_c, index)

    coder.extrinsic('Manipulator_Dynamics');
    qdot = zeros(3, 1);
    pdot = zeros(3, 1);
    [qdot, pdot] = Manipulator_Dynamics(q, p, tau_l, tau_c, index);

== matlab function Model_2Systems_Manipulators/Manipulator1/Hamiltonian Plant/r-passivity Validation/MATLAB Function ==
  data: Vdot output; q input; qdot input; p input; pdot input; r input; tau_kv input; y_d input; index input; V output; Vr0 parameter; S output; Kv parameter
function [Vdot, V, S] = fcn(q, qdot, p, pdot, r, tau_kv, y_d, index, Vr0, Kv)

    coder.extrinsic('R_Validation');
    V = zeros(1,1); Vdot = 0; S = 0;
    [V, Vdot, S] = R_Validation(q, qdot,p, pdot, r, tau_kv, y_d, Kv, index);
    V = V - Vr0;
end

== matlab function Model_2Systems_Manipulators/Manipulator1/Levenberg Compensation ==
  data: q input; tau_k input; z_dot input; tau_c output; index input
function tau_c  = Pre(q, tau_k, z_dot, index)

    coder.extrinsic('Manipulator_Pre');
    tau_c = zeros(2,1);
    [tau_c] = Manipulator_Pre(q, tau_k, z_dot, index);
end

== matlab function Model_2Systems_Manipulators/Edge 1/Formation Retrieval ==
  data: i input; r_ij output; j input; R input
function r_ij = get_rij(i, j, R)
    %r_ij = zeros(2,1);
    r_ij = [R((i - 1)*2 + 1, j);R(2*i, j)];
end

== matlab function Model_2Systems_Manipulators/Manipulator2/Hamiltonian Plant/r-passivity Validation/MATLAB Function ==
  data: Vdot output; q input; qdot input; p input; pdot input; r input; tau_kv input; y_d input; index input; V output; Vr0 parameter; S output; Kv parameter
function [Vdot, V, S] = fcn(q, qdot, p, pdot, r, tau_kv, y_d, index, Vr0, Kv)

    coder.extrinsic('R_Validation');
    V = zeros(1,1); Vdot = 0; S = 0;
    [V, Vdot, S] = R_Validation(q, qdot,p, pdot, r, tau_kv, y_d, Kv, index);
    V = V - Vr0;
end

== matlab function Model_2Systems_Manipulators/Manipulator2/Levenberg Compensation ==
  data: q input; tau_k input; z_dot input; tau_c output; index input
function tau_c  = Pre(q, tau_k, z_dot, index)

    coder.extrinsic('Manipulator_Pre');
    tau_c = zeros(2,1);
    [tau_c] = Manipulator_Pre(q, tau_k, z_dot, index);
end

== matlab function Model_2Systems_Manipulators/Manipulator2/MATLAB Function1 ==
  data: p input; q input; tau output; tau_fb output; index input
function [tau, tau_fb] = LocalControl(p, q, index)
    

coder.extrinsic('Manipulator_Control');
tau = zeros(3, 1);
tau_fb = zeros(2, 1);
tau_Kv = zeros(2, 1);
[tau, tau_fb] = Manipulator_Control(q, p, index);

== matlab function Model_2Systems_Manipulators/Manipulator1/MATLAB Function1 ==
  data: p input; q input; tau output; tau_fb output; index input
function [tau, tau_fb] = LocalControl(p, q, index)
    

coder.extrinsic('Manipulator_Control');
tau = zeros(3, 1);
tau_fb = zeros(2, 1);
tau_Kv = zeros(2, 1);
[tau, tau_fb] = Manipulator_Control(q, p, index);

== matlab function Model_2Systems_Manipulators/Manipulator3/Hamiltonian Plant/MATLAB Function1 ==
  data: q input; z output; p input; r output; index input; z_dot output
function [z, r, z_dot] = toz(q, p, index)

    coder.extrinsic('Manipulator_z');
    z = zeros(2, 1);
    r = zeros(2, 1);
    z_dot = zeros(2, 1);
    [z, r, z_dot] = Manipulator_z(q, p, index);

== matlab function Model_2Systems_Manipulators/Manipulator3/Hamiltonian Plant/MATLAB Function2 ==
  data: q input; qdot output; p input; tau_l input; pdot output; tau_c input; index input
function [qdot, pdot] = fcn(q, p, tau_l, tau_c, index)

    coder.extrinsic('Manipulator_Dynamics');
    qdot = zeros(3, 1);
    pdot = zeros(3, 1);
    [qdot, pdot] = Manipulator_Dynamics(q, p, tau_l, tau_c, index);

== matlab function Model_2Systems_Manipulators/Manipulator3/Hamiltonian Plant/r-passivity Validation/MATLAB Function ==
  data: Vdot output; q input; qdot input; p input; pdot input; r input; tau_kv input; y_d input; index input; V output; Vr0 parameter; Vcomp output; Kv parameter
function [Vdot, V, Vcomp] = fcn(q, qdot, p, pdot, r, tau_kv, y_d, index, Vr0, Kv)

    coder.extrinsic('R_Validation');
    V = zeros(1,1); Vdot = 0; Vcomp = zeros(1,1);
    [V, Vdot, Vcomp] = R_Validation(q, qdot,p, pdot, r, tau_kv, y_d, Kv, index);
    V = V - Vr0;
end

== matlab function Model_2Systems_Manipulators/Manipulator3/Levenberg Compensation ==
  data: q input; tau_k input; tau_c output; index input
function tau_c  = Pre(q, tau_k, index)

    coder.extrinsic('Manipulator_Pre');
    tau_c = zeros(2,1);
    [tau_c] = Manipulator_Pre(q, tau_k, index);
end

== matlab function Model_2Systems_Manipulators/Manipulator3/MATLAB Function1 ==
  data: p input; q input; tau output; tau_fb output; index input
function [tau, tau_fb] = LocalControl(p, q, index)
    

coder.extrinsic('Manipulator_Control');
tau = zeros(3, 1);
tau_fb = zeros(2, 1);
tau_Kv = zeros(2, 1);
[tau, tau_fb] = Manipulator_Control(q, p, index);

== matlab function Model_2Systems_Manipulators/UAV2/Hamiltonian Plant/MATLAB Function1 ==
  data: q input; z output; p input; r output; index input; z_dot output
function [z, r, z_dot] = toz(q, p, index)

    coder.extrinsic('UAV_z');
    z = zeros(2, 1);
    r = zeros(2, 1);
    z_dot = zeros(2, 1);
    [z, r, z_dot] = UAV_z(q, p, index);

== matlab function Model_2Systems_Manipulators/UAV2/Hamiltonian Plant/MATLAB Function2 ==
  data: q input; qdot output; p input; tau_l input; pdot output; tau_c input; index input
function [qdot, pdot] = fcn(q, p, tau_l, tau_c, index)

    coder.extrinsic('UAV_Dynamics');
    qdot = zeros(3, 1);
    pdot = zeros(3, 1);
    [qdot, pdot] = UAV_Dynamics(q, p, tau_l, tau_c, index);

== matlab function Model_2Systems_Manipulators/UAV/Hamiltonian Plant/MATLAB Function ==
  data: q input; r input; index input; V output; Vr0 parameter
function V = fcn(q, r, index, Vr0)

%     coder.extrinsic('R_Validation');
%     V = 0;
%     [V] = R_Validation(q, r, index);
%     V = V - Vr0;
V = 0;
end

== matlab function Model_2Systems_Manipulators/UAV/Hamiltonian Plant/MATLAB Function1 ==
  data: q input; z output; p input; r output; index input; y_d output
function [z, r, y_d] = toz(q, p, index)

    coder.extrinsic('UAV_z');
    z = zeros(2, 1);
    r = zeros(2, 1);  
    y_d = zeros(2, 1);
    [z, r, y_d] = UAV_z(q, p, index);

== matlab function Model_2Systems_Manipulators/UAV/Hamiltonian Plant/MATLAB Function2 ==
  data: q input; qdot output; p input; tau_l input; pdot output; tau_c input; index input
function [qdot, pdot] = fcn(q, p, tau_l, tau_c, index)

    coder.extrinsic('UAV_Dynamics');
    qdot = zeros(3, 1);
    pdot = zeros(3, 1);
    [qdot, pdot] = UAV_Dynamics(q, p, tau_l, tau_c, index);

== matlab function Model_2Systems_Manipulators/UAV/MATLAB Function1 ==
  data: p input; q input; tau output; tau_fb output; index input
function [tau, tau_fb] = LocalControl(p, q, index)
    

coder.extrinsic('UAV_Control');
tau = zeros(2, 1);
tau_fb = zeros(2, 1);
[tau, tau_fb] = UAV_Control(q, p, index);

== matlab function Model_2Systems_Manipulators/UAV2/Hamiltonian Plant/r-passivity Validation/MATLAB Function ==
  data: Vdot output; q input; qdot input; p input; pdot input; r input; tau_kv input; y_d input; index input; V output; Vr0 parameter; S output; Kv parameter
function [Vdot, V, S] = fcn(q, qdot, p, pdot, r, tau_kv, y_d, index, Vr0, Kv)

    coder.extrinsic('R_Validation');
    V = zeros(1,1); Vdot = 0; S = 0;
    [V, Vdot, S] = R_Validation(q, qdot,p, pdot, r, tau_kv, y_d, Kv, index);
    V = V - Vr0;
end

== matlab function Model_2Systems_Manipulators/UAV2/Levenberg Compensation ==
  data: q input; tau_k input; z_dot input; tau_c output; index input
function tau_c  = Pre(q, tau_k, z_dot, index)

    coder.extrinsic('Manipulator_Pre');
    tau_c = zeros(2,1);
    [tau_c] = Manipulator_Pre(q, tau_k, z_dot, index);
end

== matlab function Model_2Systems_Manipulators/UAV2/MATLAB Function1 ==
  data: p input; q input; tau output; tau_fb output; index input
function [tau, tau_fb] = LocalControl(p, q, index)
    

coder.extrinsic('UAV_Control');
tau = zeros(2, 1);
tau_fb = zeros(2, 1);
tau_Kv = zeros(2, 1);
[tau, tau_fb] = UAV_Control(q, p, index);

== matlab function Model_2Systems_Manipulators/UAV2/MATLAB Function ==
  data: q input; beta output; p input; tau_c input
function beta  = fb_optimise(q, p, tau_c)

y = u;
